simulink library "MantaFSController_cl"  (R2020a)
settings: Solver=VariableStepAuto  StartTime=0.0  StopTime=10.0  RelTol=1e-3
undefined symbols (not defined in the file or in its folder): a, env, FLIGHTCONTROLLER, fltCtrl, initializeBussesFromBlock, pthCtrl1, pthCtrl2, slfCtrl, thr, vhcl, wnch
libraries: simulink x21, angleBtw2Vecs_ul x9, pathGeometry_ul x6, filteredPIDController_ul x5, ctrlAllocMatrix_cl x4, tanFrameProjection_ul x4, vectorNormalizer_ul x4, velocityAngle_ul x4, filteredPIDControllerAWGS_ul x3, eulAng2RotMat_ul x3, vrlib x3, alphaBeta_ul x3
(part 3 of 3)

== system MantaFSController_cl/MantaFSController/xcurrent-lemOfBooth/pathFollowingControllerManta/courseFollowManta/GoldenSectionPathSearch/GoldenSectionSimulink/Subsystem1 ==
  In1 : Inport
  In2 : Inport  Port=2
  In3 : Inport  Port=3
  pathGeometry : pathGeometry_ul/pathGeometry  SystemSampleTime=-1  Latency=0  AutoFrameSizeCalculation=off
  Out1 : Outport  VectorParamsAs1DForOutWhenUnconnected=off
  Out2 : Outport  Port=2  VectorParamsAs1DForOutWhenUnconnected=off
  wires:
  pathGeometry/2 -> Out2/1
  In1/1 -> pathGeometry/1
  In3/1 -> pathGeometry/3
  pathGeometry/1 -> Out1/1
  In2/1 -> pathGeometry/2

== matlab function MantaFSController_cl/MantaFSController/non-xcurrent/LaRController/winchController/MATLAB Function1 ==
  data: thrLength input; elevationSP output; elevSP1 parameter; elevSP2 parameter
function elevationSP = fcn(thrLength,elevSP1, elevSP2)

if thrLength > 95
    elevationSP = elevSP1;
else
    elevationSP = elevSP2;
end

== matlab function MantaFSController_cl/MantaFSController/non-xcurrent/LaRController/winchController/MATLAB Function ==
  data: thrLength input; thrTension input; posAng input; Ctrl output; eulAng input; coneWidth parameter; leash parameter; spd parameter; elevSP input
function Ctrl  = fcn(thrLength, thrTension, posAng, eulAng, coneWidth, leash, spd, elevSP)

roll = eulAng(1)*180/pi;                                %   deg - Roll angle 
% pitch = eulAng(2)*180/pi;                               %   deg - Pitch angle 
% yaw = eulAng(3)*180/pi;                                 %   deg - Yaw angle 

elevationAngle = posAng(1);                             %   deg - Elevation angle 
elevationError = abs(elevSP-elevationAngle);            %   deg - Elevation angle error 
% if thrLength < 100
%     spd = spd;
% end
nomWidth = coneWidth/2;                                 %   deg - Width of elevation cone where nominal speed is allowed
x = [nomWidth coneWidth];
y = [-spd 0];
m = (y(2)-y(1))/(x(2)-x(1));

thrErr = thrLength-leash;                               %   m - Tether length error 

if thrErr < 1
    gain = 0.01*thrErr+0.5;
else
    gain = 1;
end

if abs(roll) > 2.5
    Ctrl = 0;
elseif elevationError <= coneWidth
    if thrErr > 1
        Ctrl = max(min(m*(elevationError-x(1))+y(1),0),-spd*gain);
    else
        Ctrl = 0;
    end
else
    Ctrl = 0;
end

== matlab function MantaFSController_cl/MantaFSController/xcurrent-lemOfBooth/pathFollowingControllerManta/courseFollowManta/GoldenSectionPathSearch/GoldenSectionMATLAB ==
  data: posVec input; sNext output; sPrev input; pathCntrPosVecGnd input; pathVarTol parameter; searchWidth parameter; geomParams input
function sNext = fcn(posVec,sPrev,pathCntrPosVecGnd, pathVarTol, searchWidth, geomParams)
% I wrote this function on 4/22/2020 when attempting to figure out some
% issues with numerical stiffness.  Turns out that althought the profiler
% was telling me the problem was with the simulink in the equivalent
% subsystem, that was a lie.  Anyways, I thought I should leave this here
% anyways just in case anyone wants to reference it.  Note that this
% implementation doesn't allow for different paths without changing
% function J below.  Which isn't great for a long term solution, so don't
% just use this as-is if you want to go to a matlab-based golden section
% implementation in the future. Also, I think there are some hard-coded
% numbers in the mask in the model, so fix that.  Finally, note that even
% though the "equivalent" simulink implementation has some inefficiencies
% that this code doesnt (as noted in the simulink implementation), there
% doesn't appear to be a siginificant difference in run times, although I
% haven't done a thorough study. -Mitchell

% phi = (sqrt(5) + 1) / 2;
% gr = 1/((1/phi)+1);
% gr = 0.618033988749895;
x1 = sPrev - searchWidth/2;
x4 = sPrev + searchWidth/2;
x2 = x4 - (x4-x1)*0.618033988749895;
x3 = x1 + (x4-x1)*0.618033988749895;
% J1 = J(x1,posVec,geomParams,pathCntrPosVecGnd);
J2 = J(x2,posVec,geomParams,pathCntrPosVecGnd);
J3 = J(x3,posVec,geomParams,pathCntrPosVecGnd);
% J4 = J(x4,posVec,geomParams,pathCntrPosVecGnd);
% JL =JFunc(xL);
% JR = JFunc(xR);
% plot([x1 x2 x3 x4],[J1 J2 J3 J4])
for ii = 1:100 
    if J2<J3
        x4 = x3;
%         J4 = J(x4,posVec,geomParams,pathCntrPosVecGnd);
        x3 = x2;
        J3 = J2;
        x2 = x4 - (x4-x1)*0.618033988749895;
        J2 = J(x2,posVec,geomParams,pathCntrPosVecGnd);
    else
        x1 = x2;
%         J1 = J(x1,posVec,geomParams,pathCntrPosVecGnd);
        x2 = x3;
        J2 = J3;
        x3 = x1 + (x4-x1)*0.618033988749895;
        J3 = J(x3,posVec,geomParams,pathCntrPosVecGnd);
    end
    if x4-x1<pathVarTol/2
        break
    end
end
sNext = mod((x4+x1)/2,1);
end

function val = J(sTest,posVec,geomParams,pathCntr)
az = atan2(posVec(2),posVec(1));
el = atan2(posVec(3),sqrt(posVec(1)^2+posVec(2)^2));
pathPosVec = lemOfBooth(sTest,geomParams,pathCntr);
azP = atan2(pathPosVec(2),pathPosVec(1));
elP = atan2(pathPosVec(3),sqrt(pathPosVec(1)^2+pathPosVec(2)^2));
val = (az-azP)^2+(el-elP)^2;
end

== matlab function MantaFSController_cl/MantaFSController/xcurrent-ellipse/pathFollowingControllerManta1/courseFollowManta/GoldenSectionPathSearch/GoldenSectionMATLAB ==
  data: posVec input; sNext output; sPrev input; pathCntrPosVecGnd input; pathVarTol parameter; searchWidth parameter; geomParams input
function sNext = fcn(posVec,sPrev,pathCntrPosVecGnd, pathVarTol, searchWidth, geomParams)
% I wrote this function on 4/22/2020 when attempting to figure out some
% issues with numerical stiffness.  Turns out that althought the profiler
% was telling me the problem was with the simulink in the equivalent
% subsystem, that was a lie.  Anyways, I thought I should leave this here
% anyways just in case anyone wants to reference it.  Note that this
% implementation doesn't allow for different paths without changing
% function J below.  Which isn't great for a long term solution, so don't
% just use this as-is if you want to go to a matlab-based golden section
% implementation in the future. Also, I think there are some hard-coded
% numbers in the mask in the model, so fix that.  Finally, note that even
% though the "equivalent" simulink implementation has some inefficiencies
% that this code doesnt (as noted in the simulink implementation), there
% doesn't appear to be a siginificant difference in run times, although I
% haven't done a thorough study. -Mitchell

% phi = (sqrt(5) + 1) / 2;
% gr = 1/((1/phi)+1);
% gr = 0.618033988749895;
x1 = sPrev - searchWidth/2;
x4 = sPrev + searchWidth/2;
x2 = x4 - (x4-x1)*0.618033988749895;
x3 = x1 + (x4-x1)*0.618033988749895;
% J1 = J(x1,posVec,geomParams,pathCntrPosVecGnd);
J2 = J(x2,posVec,geomParams,pathCntrPosVecGnd);
J3 = J(x3,posVec,geomParams,pathCntrPosVecGnd);
% J4 = J(x4,posVec,geomParams,pathCntrPosVecGnd);
% JL =JFunc(xL);
% JR = JFunc(xR);
% plot([x1 x2 x3 x4],[J1 J2 J3 J4])
for ii = 1:100 
    if J2<J3
        x4 = x3;
%         J4 = J(x4,posVec,geomParams,pathCntrPosVecGnd);
        x3 = x2;
        J3 = J2;
        x2 = x4 - (x4-x1)*0.618033988749895;
        J2 = J(x2,posVec,geomParams,pathCntrPosVecGnd);
    else
        x1 = x2;
%         J1 = J(x1,posVec,geomParams,pathCntrPosVecGnd);
        x2 = x3;
        J2 = J3;
        x3 = x1 + (x4-x1)*0.618033988749895;
        J3 = J(x3,posVec,geomParams,pathCntrPosVecGnd);
    end
    if x4-x1<pathVarTol/2
        break
    end
end
sNext = mod((x4+x1)/2,1);
end

function val = J(sTest,posVec,geomParams,pathCntr)
az = atan2(posVec(2),posVec(1));
el = atan2(posVec(3),sqrt(posVec(1)^2+posVec(2)^2));
pathPosVec = lemOfBooth(sTest,geomParams,pathCntr);
azP = atan2(pathPosVec(2),pathPosVec(1));
elP = atan2(pathPosVec(3),sqrt(pathPosVec(1)^2+pathPosVec(2)^2));
val = (az-azP)^2+(el-elP)^2;
end
